simulink library "cool_simple_retOnly_std"  (R2016a)
settings: Solver=VariableStepAuto  StartTime=0.0  StopTime=10.0  RelTol=1e-3
undefined symbols (not defined in the file): sMP
settings Model: Creator=JEKREMS  LastModifiedBy=JEKREMS
settings GRTTargetCC: GeneratePreprocessorConditionals=Use local settings

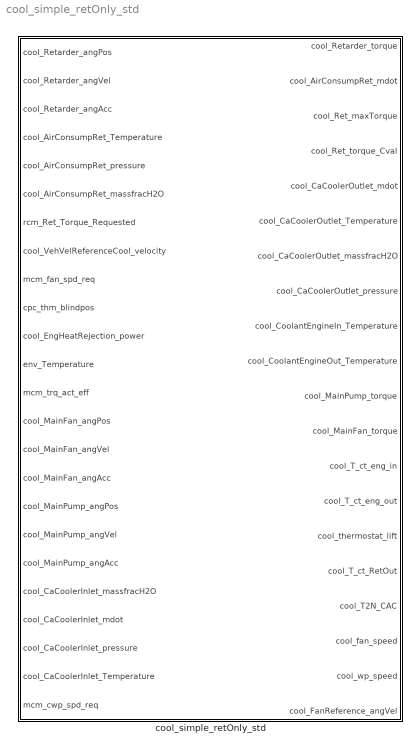
== system cool_simple_retOnly_std ==
  cool_simple_retOnly_std : Subsystem  mask{prm_to_disp=[1..10], sfcnParam1=sMP.phys.cool.fan.x_fan_rpm_schlepp, sfcnParam2=sMP.phys.cool.fan.y_fan_M_schlepp, sfcnParam3=sMP.phys.cool.out.cool_CaCoolerOutlet_Temperature, sfcnParam4=sMP.phys.cool.out.cool_CoolantEngineIn_Temperature, sfcnParam5=sMP.phys.cool.out.cool_CoolantEngineOut_Temperature, sfcnParam6=sMP.phys.cool.out.cool_T2N_CAC, sfcnParam7=sMP.phys.cool.out.cool_T_ct_RetOut, sfcnParam8=sMP.phys.cool.out.cool_T_ct_eng_in, sfcnParam9=sMP.phys.cool.out.cool_T_ct_eng_out, sfcnParam10=sMP.phys.cool.ret.x_ret_rpm, sfcnParam11=sMP.phys.cool.ret.x_ret_rpm_schlepp, sfcnParam12=sMP.phys.cool.ret.y_ret_M_max, sfcnParam13=sMP.phys.cool.ret.y_ret_M_schlepp}
      mask prompts: prm_to_disp "Display S-function Parameters:"; sfcnParam1 "fan_x_fan_rpm_schlepp:"; sfcnParam2 "fan_y_fan_M_schlepp:"; sfcnParam3 "out_cool_CaCoolerOutlet_Temperature:"; sfcnParam4 "out_cool_CoolantEngineIn_Temperature:"; sfcnParam5 "out_cool_CoolantEngineOut_Temperature:"; sfcnParam6 "out_cool_T2N_CAC:"; sfcnParam7 "out_cool_T_ct_RetOut:"; sfcnParam8 "out_cool_T_ct_eng_in:"; sfcnParam9 "out_cool_T_ct_eng_out:"; sfcnParam10 "ret_x_ret_rpm:"; sfcnParam11 "ret_x_ret_rpm_schlepp:"; sfcnParam12 "ret_y_ret_M_max:"; sfcnParam13 "ret_y_ret_M_schlepp:"
      mask help: Simulink:masks:GenSFuncDesc_MD
      mask Help: eval('feval(''rtwprivate'',''rtwhelpview'',''rtw_sfcn_block'')');
      mask TypeOptions prm_to_disp: [1..10] | [11..13]
      mask Callback prm_to_disp: slmaskprmdispcntrl(gcbh)

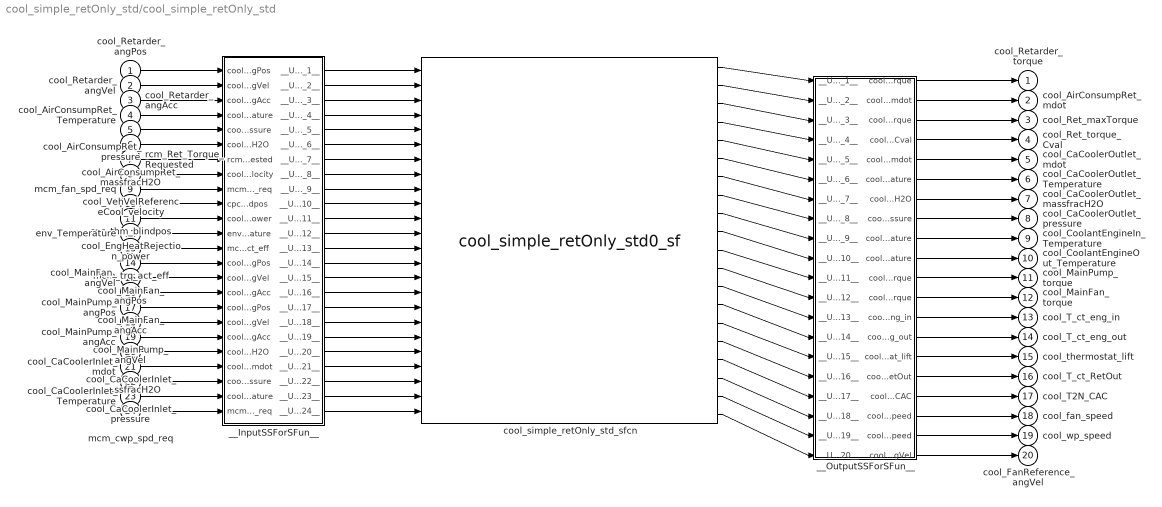
== system cool_simple_retOnly_std/cool_simple_retOnly_std ==
  cool_Retarder_angPos : Inport
  cool_Retarder_angVel : Inport  Port=2
  cool_Retarder_angAcc : Inport  Port=3
  cool_AirConsumpRet_Temperature : Inport  Port=4
  cool_AirConsumpRet_pressure : Inport  Port=5
  cool_AirConsumpRet_massfracH2O : Inport  Port=6
  rcm_Ret_Torque_Requested : Inport  Port=7
  cool_VehVelReferenceCool_velocity : Inport  Port=8
  mcm_fan_spd_req : Inport  Port=9
  cpc_thm_blindpos : Inport  Port=10
  cool_EngHeatRejection_power : Inport  Port=11
  env_Temperature : Inport  Port=12
  mcm_trq_act_eff : Inport  Port=13
  cool_MainFan_angPos : Inport  Port=14
  cool_MainFan_angVel : Inport  Port=15
  cool_MainFan_angAcc : Inport  Port=16
  cool_MainPump_angPos : Inport  Port=17
  cool_MainPump_angVel : Inport  Port=18
  cool_MainPump_angAcc : Inport  Port=19
  cool_CaCoolerInlet_massfracH2O : Inport  Port=20
  cool_CaCoolerInlet_mdot : Inport  Port=21
  cool_CaCoolerInlet_pressure : Inport  Port=22
  cool_CaCoolerInlet_Temperature : Inport  Port=23
  mcm_cwp_spd_req : Inport  Port=24
  __InputSSForSFun__ : Subsystem
  __OutputSSForSFun__ : Subsystem
  cool_simple_retOnly_std_sfcn : S-Function  FunctionName=cool_simple_retOnly_std0_sf  Parameters=sfcnParam1, sfcnParam2, sfcnParam3, sfcnParam4, sfcnParam5, sfcnParam6, sfcnParam7, sfcnParam8, sfcnParam9, sfcnParam10, sfcnParam11, sfcnParam12, sfcnParam13  SFunctionModules=""  SFunctionDeploymentMode=off  EnableBusSupport=off  mask{rtw_sf_name=cool_simple_retOnly_std0_sf, showVar=off, prm_to_disp=[1..10], sfcnParam1=sfcnParam1, sfcnParam2=sfcnParam2, sfcnParam3=sfcnParam3, sfcnParam4=sfcnParam4, sfcnParam5=sfcnParam5, sfcnParam6=sfcnParam6, sfcnParam7=sfcnParam7, sfcnParam8=sfcnParam8, sfcnParam9=sfcnParam9, sfcnParam10=sfcnParam10, sfcnParam11=sfcnParam11, sfcnParam12=sfcnParam12, sfcnParam13=sfcnParam13}
      mask prompts: rtw_sf_name "Simulink:masks:GenSFuncName_MP"; showVar "Simulink:masks:GenSFuncShowModuleList_MP"; prm_to_disp "Display S-function Parameters:"; sfcnParam1 "sMP_phys_cool_fan_x_fan_rpm_schlepp:"; sfcnParam2 "sMP_phys_cool_fan_y_fan_M_schlepp:"; sfcnParam3 "sMP_phys_cool_out_cool_CaCoolerOutlet_Temperature:"; sfcnParam4 "sMP_phys_cool_out_cool_CoolantEngineIn_Temperature:"; sfcnParam5 "sMP_phys_cool_out_cool_CoolantEngineOut_Temperature:"; sfcnParam6 "sMP_phys_cool_out_cool_T2N_CAC:"; sfcnParam7 "sMP_phys_cool_out_cool_T_ct_RetOut:"; sfcnParam8 "sMP_phys_cool_out_cool_T_ct_eng_in:"; sfcnParam9 "sMP_phys_cool_out_cool_T_ct_eng_out:"; sfcnParam10 "sMP_phys_cool_ret_x_ret_rpm:"; sfcnParam11 "sMP_phys_cool_ret_x_ret_rpm_schlepp:"; sfcnParam12 "sMP_phys_cool_ret_y_ret_M_max:"; sfcnParam13 "sMP_phys_cool_ret_y_ret_M_schlepp:"
      mask help: Simulink:masks:GenSFuncDesc_MD
      mask init:
      | displist = '';
      | if ~strcmp(get_param(gcb, 'FunctionName'), rtw_sf_name);
      |   set_param(gcb, 'FunctionName', rtw_sf_name);
      | end
      | % Check if we are generating code
      | rtw_mode = false;
      | if strcmpi(get_param(bdroot(gcb),'SimulationStatus'),'Initializing')
      | 	rtw_mode = strcmpi(get_param(bdroot(gcb),'BuildingRTWCode'),'on') && ...
      | 		~strcmpi(get_param(bdroot(gcb),'TargetStyle'),'SimulationTarget');
      | end
      | if showVar || rtw_mode
      | 	if exist('rtwsfunc') == 2 | exist('rtwsfunc') == 6
      | 		tmplist = rtwsfunc(rtw_sf_name,gcb);
      | 		tmplist = DAStudio.message('Simulink:masks:GenSFuncListOfModules_IC', tmplist);
      | 	elseif showVar
      | 		tmplist1 = DAStudio.message('Simulink:masks:GenSFuncListOfModules_IC', '');
      |         tmplist2 = DAStudio.message('Simulink:masks:GenSFuncNotLicensed_IC');
      |         tmplist = [tmplist1 tmplist2];
      |  	end
      | end
      | if showVar
      |   displist = tmplist;
      | end
      settings: CopyFcn=|
      | if ~strcmp(get_param(gcb,'Linkstatus'),'none') && ...
      | ~strcmp(get_param(gcb,'Linkstatus'),'implicit')
      |   set_param(gcb,'LinkStatus','none');
      | end
      mask Help: eval('feval(''rtwprivate'',''rtwhelpview'',''rtw_sfcn_block'')');
      mask TypeOptions prm_to_disp: [1..10] | [11..13]
      mask Callback prm_to_disp: slmaskprmdispcntrl(gcbh)
      mask Display:
      | port_label('input',1,'cool_Retarder_angPos');
      | port_label('input',2,'cool_Retarder_angVel');
      | port_label('input',3,'cool_Retarder_angAcc');
      | port_label('input',4,'cool_AirConsumpRet_Temperature');
      | port_label('input',5,'cool_AirConsumpRet_pressure');
      | port_label('input',6,'cool_AirConsumpRet_massfracH2O');
      | port_label('input',7,'rcm_Ret_Torque_Requested');
      | port_label('input',8,'cool_VehVelReferenceCool_velocity');
      | port_label('input',9,'mcm_fan_spd_req');
      | port_label('input',10,'cpc_thm_blindpos');
      | port_label('input',11,'cool_EngHeatRejection_power');
      | port_label('input',12,'env_Temperature');
      | port_label('input',13,'mcm_trq_act_eff');
      | port_label('input',14,'cool_MainFan_angPos');
      | port_label('input',15,'cool_MainFan_angVel');
      | port_label('input',16,'cool_MainFan_angAcc');
      | port_label('input',17,'cool_MainPump_angPos');
      | port_label('input',18,'cool_MainPump_angVel');
      | port_label('input',19,'cool_MainPump_angAcc');
      | port_label('input',20,'cool_CaCoolerInlet_massfracH2O');
      | port_label('input',21,'cool_CaCoolerInlet_mdot');
      | port_label('input',22,'cool_CaCoolerInlet_pressure');
      | port_label('input',23,'cool_CaCoolerInlet_Temperature');
      | port_label('input',24,'mcm_cwp_spd_req');
      | port_label('output',1,'cool_Retarder_torque');
      | port_label('output',2,'cool_AirConsumpRet_mdot');
      | port_label('output',3,'cool_Ret_maxTorque');
      | port_label('output',4,'cool_Ret_torque_Cval');
      | port_label('output',5,'cool_CaCoolerOutlet_mdot');
      | port_label('output',6,'cool_CaCoolerOutlet_Temperature');
      | port_label('output',7,'cool_CaCoolerOutlet_massfracH2O');
      | port_label('output',8,'cool_CaCoolerOutlet_pressure');
      | port_label('output',9,'cool_CoolantEngineIn_Temperature');
      | port_label('output',10,'cool_CoolantEngineOut_Temperature');
      | port_label('output',11,'cool_MainPump_torque');
      | port_label('output',12,'cool_MainFan_torque');
      | port_label('output',13,'cool_T_ct_eng_in');
      | port_label('output',14,'cool_T_ct_eng_out');
      | port_label('output',15,'cool_thermostat_lift');
      | port_label('output',16,'cool_T_ct_RetOut');
      | port_label('output',17,'cool_T2N_CAC');
      | port_label('output',18,'cool_fan_speed');
      | port_label('output',19,'cool_wp_speed');
      | port_label('output',20,'cool_FanReference_angVel');
  cool_Retarder_torque : Outport
  cool_AirConsumpRet_mdot : Outport  Port=2
  cool_Ret_maxTorque : Outport  Port=3
  cool_Ret_torque_Cval : Outport  Port=4
  cool_CaCoolerOutlet_mdot : Outport  Port=5
  cool_CaCoolerOutlet_Temperature : Outport  Port=6
  cool_CaCoolerOutlet_massfracH2O : Outport  Port=7
  cool_CaCoolerOutlet_pressure : Outport  Port=8
  cool_CoolantEngineIn_Temperature : Outport  Port=9
  cool_CoolantEngineOut_Temperature : Outport  Port=10
  cool_MainPump_torque : Outport  Port=11
  cool_MainFan_torque : Outport  Port=12
  cool_T_ct_eng_in : Outport  Port=13
  cool_T_ct_eng_out : Outport  Port=14
  cool_thermostat_lift : Outport  Port=15
  cool_T_ct_RetOut : Outport  Port=16
  cool_T2N_CAC : Outport  Port=17
  cool_fan_speed : Outport  Port=18
  cool_wp_speed : Outport  Port=19
  cool_FanReference_angVel : Outport  Port=20
  wires:
  __OutputSSForSFun__/20(cool_FanReference_angVel) -> cool_FanReference_angVel/1
  __OutputSSForSFun__/19(cool_wp_speed) -> cool_wp_speed/1
  __OutputSSForSFun__/18(cool_fan_speed) -> cool_fan_speed/1
  __OutputSSForSFun__/17(cool_T2N_CAC) -> cool_T2N_CAC/1
  __OutputSSForSFun__/16(cool_T_ct_RetOut) -> cool_T_ct_RetOut/1
  __OutputSSForSFun__/15(cool_thermostat_lift) -> cool_thermostat_lift/1
  __OutputSSForSFun__/14(cool_T_ct_eng_out) -> cool_T_ct_eng_out/1
  __OutputSSForSFun__/13(cool_T_ct_eng_in) -> cool_T_ct_eng_in/1
  __OutputSSForSFun__/12(cool_MainFan_torque) -> cool_MainFan_torque/1
  __OutputSSForSFun__/11(cool_MainPump_torque) -> cool_MainPump_torque/1
  __OutputSSForSFun__/10(cool_CoolantEngineOut_Temperature) -> cool_CoolantEngineOut_Temperature/1
  __OutputSSForSFun__/9(cool_CoolantEngineIn_Temperature) -> cool_CoolantEngineIn_Temperature/1
  __OutputSSForSFun__/8(cool_CaCoolerOutlet_pressure) -> cool_CaCoolerOutlet_pressure/1
  __OutputSSForSFun__/7(cool_CaCoolerOutlet_massfracH2O) -> cool_CaCoolerOutlet_massfracH2O/1
  __OutputSSForSFun__/6(cool_CaCoolerOutlet_Temperature) -> cool_CaCoolerOutlet_Temperature/1
  __OutputSSForSFun__/5(cool_CaCoolerOutlet_mdot) -> cool_CaCoolerOutlet_mdot/1
  __OutputSSForSFun__/4(cool_Ret_torque_Cval) -> cool_Ret_torque_Cval/1
  __OutputSSForSFun__/3(cool_Ret_maxTorque) -> cool_Ret_maxTorque/1
  __OutputSSForSFun__/2(cool_AirConsumpRet_mdot) -> cool_AirConsumpRet_mdot/1
  __OutputSSForSFun__/1(cool_Retarder_torque) -> cool_Retarder_torque/1
  cool_simple_retOnly_std_sfcn/20 -> __OutputSSForSFun__/20(__UniqueInportName__20__)
  cool_simple_retOnly_std_sfcn/19 -> __OutputSSForSFun__/19(__UniqueInportName__19__)
  cool_simple_retOnly_std_sfcn/18 -> __OutputSSForSFun__/18(__UniqueInportName__18__)
  cool_simple_retOnly_std_sfcn/17 -> __OutputSSForSFun__/17(__UniqueInportName__17__)
  cool_simple_retOnly_std_sfcn/16 -> __OutputSSForSFun__/16(__UniqueInportName__16__)
  cool_simple_retOnly_std_sfcn/15 -> __OutputSSForSFun__/15(__UniqueInportName__15__)
  cool_simple_retOnly_std_sfcn/14 -> __OutputSSForSFun__/14(__UniqueInportName__14__)
  cool_simple_retOnly_std_sfcn/13 -> __OutputSSForSFun__/13(__UniqueInportName__13__)
  cool_simple_retOnly_std_sfcn/12 -> __OutputSSForSFun__/12(__UniqueInportName__12__)
  cool_simple_retOnly_std_sfcn/11 -> __OutputSSForSFun__/11(__UniqueInportName__11__)
  cool_simple_retOnly_std_sfcn/10 -> __OutputSSForSFun__/10(__UniqueInportName__10__)
  cool_simple_retOnly_std_sfcn/9 -> __OutputSSForSFun__/9(__UniqueInportName__9__)
  cool_simple_retOnly_std_sfcn/8 -> __OutputSSForSFun__/8(__UniqueInportName__8__)
  cool_simple_retOnly_std_sfcn/7 -> __OutputSSForSFun__/7(__UniqueInportName__7__)
  cool_simple_retOnly_std_sfcn/6 -> __OutputSSForSFun__/6(__UniqueInportName__6__)
  cool_simple_retOnly_std_sfcn/5 -> __OutputSSForSFun__/5(__UniqueInportName__5__)
  cool_simple_retOnly_std_sfcn/4 -> __OutputSSForSFun__/4(__UniqueInportName__4__)
  cool_simple_retOnly_std_sfcn/3 -> __OutputSSForSFun__/3(__UniqueInportName__3__)
  cool_simple_retOnly_std_sfcn/2 -> __OutputSSForSFun__/2(__UniqueInportName__2__)
  cool_simple_retOnly_std_sfcn/1 -> __OutputSSForSFun__/1(__UniqueInportName__1__)
  __InputSSForSFun__/24(__UniqueOutportName__24__) -> cool_simple_retOnly_std_sfcn/24
  __InputSSForSFun__/23(__UniqueOutportName__23__) -> cool_simple_retOnly_std_sfcn/23
  __InputSSForSFun__/22(__UniqueOutportName__22__) -> cool_simple_retOnly_std_sfcn/22
  __InputSSForSFun__/21(__UniqueOutportName__21__) -> cool_simple_retOnly_std_sfcn/21
  __InputSSForSFun__/20(__UniqueOutportName__20__) -> cool_simple_retOnly_std_sfcn/20
  __InputSSForSFun__/19(__UniqueOutportName__19__) -> cool_simple_retOnly_std_sfcn/19
  __InputSSForSFun__/18(__UniqueOutportName__18__) -> cool_simple_retOnly_std_sfcn/18
  __InputSSForSFun__/17(__UniqueOutportName__17__) -> cool_simple_retOnly_std_sfcn/17
  __InputSSForSFun__/16(__UniqueOutportName__16__) -> cool_simple_retOnly_std_sfcn/16
  __InputSSForSFun__/15(__UniqueOutportName__15__) -> cool_simple_retOnly_std_sfcn/15
  __InputSSForSFun__/14(__UniqueOutportName__14__) -> cool_simple_retOnly_std_sfcn/14
  __InputSSForSFun__/13(__UniqueOutportName__13__) -> cool_simple_retOnly_std_sfcn/13
  __InputSSForSFun__/12(__UniqueOutportName__12__) -> cool_simple_retOnly_std_sfcn/12
  __InputSSForSFun__/11(__UniqueOutportName__11__) -> cool_simple_retOnly_std_sfcn/11
  __InputSSForSFun__/10(__UniqueOutportName__10__) -> cool_simple_retOnly_std_sfcn/10
  __InputSSForSFun__/9(__UniqueOutportName__9__) -> cool_simple_retOnly_std_sfcn/9
  __InputSSForSFun__/8(__UniqueOutportName__8__) -> cool_simple_retOnly_std_sfcn/8
  __InputSSForSFun__/7(__UniqueOutportName__7__) -> cool_simple_retOnly_std_sfcn/7
  __InputSSForSFun__/6(__UniqueOutportName__6__) -> cool_simple_retOnly_std_sfcn/6
  __InputSSForSFun__/5(__UniqueOutportName__5__) -> cool_simple_retOnly_std_sfcn/5
  __InputSSForSFun__/4(__UniqueOutportName__4__) -> cool_simple_retOnly_std_sfcn/4
  __InputSSForSFun__/3(__UniqueOutportName__3__) -> cool_simple_retOnly_std_sfcn/3
  __InputSSForSFun__/2(__UniqueOutportName__2__) -> cool_simple_retOnly_std_sfcn/2
  __InputSSForSFun__/1(__UniqueOutportName__1__) -> cool_simple_retOnly_std_sfcn/1
  mcm_cwp_spd_req/1 -> __InputSSForSFun__/24(mcm_cwp_spd_req)
  cool_CaCoolerInlet_Temperature/1 -> __InputSSForSFun__/23(cool_CaCoolerInlet_Temperature)
  cool_CaCoolerInlet_pressure/1 -> __InputSSForSFun__/22(cool_CaCoolerInlet_pressure)
  cool_CaCoolerInlet_mdot/1 -> __InputSSForSFun__/21(cool_CaCoolerInlet_mdot)
  cool_CaCoolerInlet_massfracH2O/1 -> __InputSSForSFun__/20(cool_CaCoolerInlet_massfracH2O)
  cool_MainPump_angAcc/1 -> __InputSSForSFun__/19(cool_MainPump_angAcc)
  cool_MainPump_angVel/1 -> __InputSSForSFun__/18(cool_MainPump_angVel)
  cool_MainPump_angPos/1 -> __InputSSForSFun__/17(cool_MainPump_angPos)
  cool_MainFan_angAcc/1 -> __InputSSForSFun__/16(cool_MainFan_angAcc)
  cool_MainFan_angVel/1 -> __InputSSForSFun__/15(cool_MainFan_angVel)
  cool_MainFan_angPos/1 -> __InputSSForSFun__/14(cool_MainFan_angPos)
  mcm_trq_act_eff/1 -> __InputSSForSFun__/13(mcm_trq_act_eff)
  env_Temperature/1 -> __InputSSForSFun__/12(env_Temperature)
  cool_EngHeatRejection_power/1 -> __InputSSForSFun__/11(cool_EngHeatRejection_power)
  cpc_thm_blindpos/1 -> __InputSSForSFun__/10(cpc_thm_blindpos)
  mcm_fan_spd_req/1 -> __InputSSForSFun__/9(mcm_fan_spd_req)
  cool_VehVelReferenceCool_velocity/1 -> __InputSSForSFun__/8(cool_VehVelReferenceCool_velocity)
  rcm_Ret_Torque_Requested/1 -> __InputSSForSFun__/7(rcm_Ret_Torque_Requested)
  cool_AirConsumpRet_massfracH2O/1 -> __InputSSForSFun__/6(cool_AirConsumpRet_massfracH2O)
  cool_AirConsumpRet_pressure/1 -> __InputSSForSFun__/5(cool_AirConsumpRet_pressure)
  cool_AirConsumpRet_Temperature/1 -> __InputSSForSFun__/4(cool_AirConsumpRet_Temperature)
  cool_Retarder_angAcc/1 -> __InputSSForSFun__/3(cool_Retarder_angAcc)
  cool_Retarder_angVel/1 -> __InputSSForSFun__/2(cool_Retarder_angVel)
  cool_Retarder_angPos/1 -> __InputSSForSFun__/1(cool_Retarder_angPos)

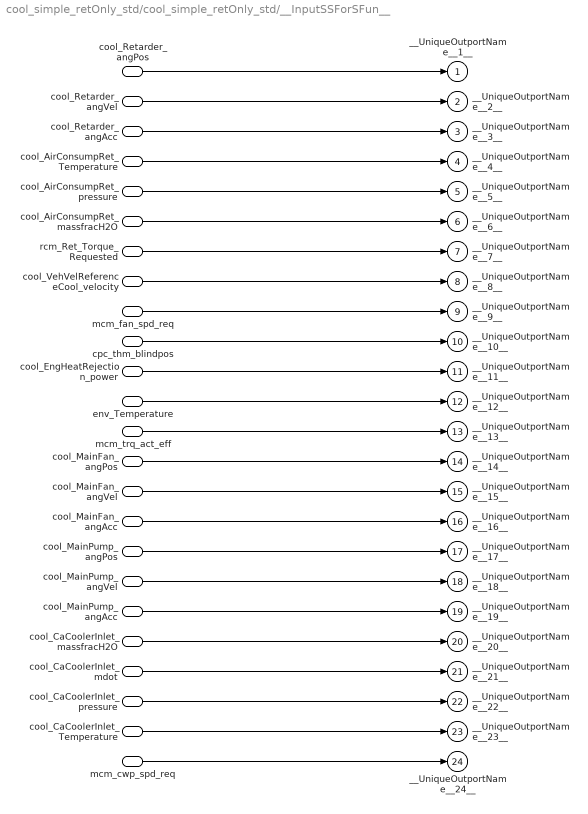
== system cool_simple_retOnly_std/cool_simple_retOnly_std/__InputSSForSFun__ ==
  cool_Retarder_angPos : Inport
  cool_Retarder_angVel : Inport  Port=2
  cool_Retarder_angAcc : Inport  Port=3
  cool_AirConsumpRet_Temperature : Inport  Port=4
  cool_AirConsumpRet_pressure : Inport  Port=5
  cool_AirConsumpRet_massfracH2O : Inport  Port=6
  rcm_Ret_Torque_Requested : Inport  Port=7
  cool_VehVelReferenceCool_velocity : Inport  Port=8
  mcm_fan_spd_req : Inport  Port=9
  cpc_thm_blindpos : Inport  Port=10
  cool_EngHeatRejection_power : Inport  Port=11
  env_Temperature : Inport  Port=12
  mcm_trq_act_eff : Inport  Port=13
  cool_MainFan_angPos : Inport  Port=14
  cool_MainFan_angVel : Inport  Port=15
  cool_MainFan_angAcc : Inport  Port=16
  cool_MainPump_angPos : Inport  Port=17
  cool_MainPump_angVel : Inport  Port=18
  cool_MainPump_angAcc : Inport  Port=19
  cool_CaCoolerInlet_massfracH2O : Inport  Port=20
  cool_CaCoolerInlet_mdot : Inport  Port=21
  cool_CaCoolerInlet_pressure : Inport  Port=22
  cool_CaCoolerInlet_Temperature : Inport  Port=23
  mcm_cwp_spd_req : Inport  Port=24
  __UniqueOutportName__1__ : Outport
  __UniqueOutportName__2__ : Outport  Port=2
  __UniqueOutportName__3__ : Outport  Port=3
  __UniqueOutportName__4__ : Outport  Port=4
  __UniqueOutportName__5__ : Outport  Port=5
  __UniqueOutportName__6__ : Outport  Port=6
  __UniqueOutportName__7__ : Outport  Port=7
  __UniqueOutportName__8__ : Outport  Port=8
  __UniqueOutportName__9__ : Outport  Port=9
  __UniqueOutportName__10__ : Outport  Port=10
  __UniqueOutportName__11__ : Outport  Port=11
  __UniqueOutportName__12__ : Outport  Port=12
  __UniqueOutportName__13__ : Outport  Port=13
  __UniqueOutportName__14__ : Outport  Port=14
  __UniqueOutportName__15__ : Outport  Port=15
  __UniqueOutportName__16__ : Outport  Port=16
  __UniqueOutportName__17__ : Outport  Port=17
  __UniqueOutportName__18__ : Outport  Port=18
  __UniqueOutportName__19__ : Outport  Port=19
  __UniqueOutportName__20__ : Outport  Port=20
  __UniqueOutportName__21__ : Outport  Port=21
  __UniqueOutportName__22__ : Outport  Port=22
  __UniqueOutportName__23__ : Outport  Port=23
  __UniqueOutportName__24__ : Outport  Port=24
  wires:
  mcm_cwp_spd_req/1 -> __UniqueOutportName__24__/1
  cool_CaCoolerInlet_Temperature/1 -> __UniqueOutportName__23__/1
  cool_CaCoolerInlet_pressure/1 -> __UniqueOutportName__22__/1
  cool_CaCoolerInlet_mdot/1 -> __UniqueOutportName__21__/1
  cool_CaCoolerInlet_massfracH2O/1 -> __UniqueOutportName__20__/1
  cool_MainPump_angAcc/1 -> __UniqueOutportName__19__/1
  cool_MainPump_angVel/1 -> __UniqueOutportName__18__/1
  cool_MainPump_angPos/1 -> __UniqueOutportName__17__/1
  cool_MainFan_angAcc/1 -> __UniqueOutportName__16__/1
  cool_MainFan_angVel/1 -> __UniqueOutportName__15__/1
  cool_MainFan_angPos/1 -> __UniqueOutportName__14__/1
  mcm_trq_act_eff/1 -> __UniqueOutportName__13__/1
  env_Temperature/1 -> __UniqueOutportName__12__/1
  cool_EngHeatRejection_power/1 -> __UniqueOutportName__11__/1
  cpc_thm_blindpos/1 -> __UniqueOutportName__10__/1
  mcm_fan_spd_req/1 -> __UniqueOutportName__9__/1
  cool_VehVelReferenceCool_velocity/1 -> __UniqueOutportName__8__/1
  rcm_Ret_Torque_Requested/1 -> __UniqueOutportName__7__/1
  cool_AirConsumpRet_massfracH2O/1 -> __UniqueOutportName__6__/1
  cool_AirConsumpRet_pressure/1 -> __UniqueOutportName__5__/1
  cool_AirConsumpRet_Temperature/1 -> __UniqueOutportName__4__/1
  cool_Retarder_angAcc/1 -> __UniqueOutportName__3__/1
  cool_Retarder_angVel/1 -> __UniqueOutportName__2__/1
  cool_Retarder_angPos/1 -> __UniqueOutportName__1__/1

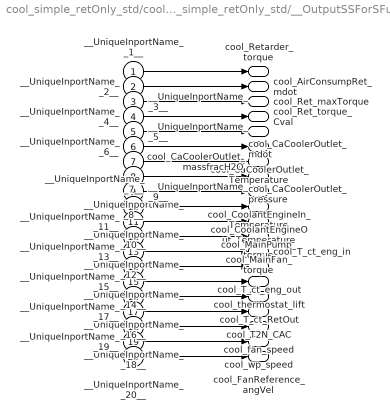
== system cool_simple_retOnly_std/cool_simple_retOnly_std/__OutputSSForSFun__ ==
  __UniqueInportName__1__ : Inport
  __UniqueInportName__2__ : Inport  Port=2
  __UniqueInportName__3__ : Inport  Port=3
  __UniqueInportName__4__ : Inport  Port=4
  __UniqueInportName__5__ : Inport  Port=5
  __UniqueInportName__6__ : Inport  Port=6
  __UniqueInportName__7__ : Inport  Port=7
  __UniqueInportName__8__ : Inport  Port=8
  __UniqueInportName__9__ : Inport  Port=9
  __UniqueInportName__10__ : Inport  Port=10
  __UniqueInportName__11__ : Inport  Port=11
  __UniqueInportName__12__ : Inport  Port=12
  __UniqueInportName__13__ : Inport  Port=13
  __UniqueInportName__14__ : Inport  Port=14
  __UniqueInportName__15__ : Inport  Port=15
  __UniqueInportName__16__ : Inport  Port=16
  __UniqueInportName__17__ : Inport  Port=17
  __UniqueInportName__18__ : Inport  Port=18
  __UniqueInportName__19__ : Inport  Port=19
  __UniqueInportName__20__ : Inport  Port=20
  cool_Retarder_torque : Outport
  cool_AirConsumpRet_mdot : Outport  Port=2
  cool_Ret_maxTorque : Outport  Port=3
  cool_Ret_torque_Cval : Outport  Port=4
  cool_CaCoolerOutlet_mdot : Outport  Port=5
  cool_CaCoolerOutlet_Temperature : Outport  Port=6
  cool_CaCoolerOutlet_massfracH2O : Outport  Port=7
  cool_CaCoolerOutlet_pressure : Outport  Port=8
  cool_CoolantEngineIn_Temperature : Outport  Port=9
  cool_CoolantEngineOut_Temperature : Outport  Port=10
  cool_MainPump_torque : Outport  Port=11
  cool_MainFan_torque : Outport  Port=12
  cool_T_ct_eng_in : Outport  Port=13
  cool_T_ct_eng_out : Outport  Port=14
  cool_thermostat_lift : Outport  Port=15
  cool_T_ct_RetOut : Outport  Port=16
  cool_T2N_CAC : Outport  Port=17
  cool_fan_speed : Outport  Port=18
  cool_wp_speed : Outport  Port=19
  cool_FanReference_angVel : Outport  Port=20
  wires:
  __UniqueInportName__20__/1 -> cool_FanReference_angVel/1
  __UniqueInportName__19__/1 -> cool_wp_speed/1
  __UniqueInportName__18__/1 -> cool_fan_speed/1
  __UniqueInportName__17__/1 -> cool_T2N_CAC/1
  __UniqueInportName__16__/1 -> cool_T_ct_RetOut/1
  __UniqueInportName__15__/1 -> cool_thermostat_lift/1
  __UniqueInportName__14__/1 -> cool_T_ct_eng_out/1
  __UniqueInportName__13__/1 -> cool_T_ct_eng_in/1
  __UniqueInportName__12__/1 -> cool_MainFan_torque/1
  __UniqueInportName__11__/1 -> cool_MainPump_torque/1
  __UniqueInportName__10__/1 -> cool_CoolantEngineOut_Temperature/1
  __UniqueInportName__9__/1 -> cool_CoolantEngineIn_Temperature/1
  __UniqueInportName__8__/1 -> cool_CaCoolerOutlet_pressure/1
  __UniqueInportName__7__/1 -> cool_CaCoolerOutlet_massfracH2O/1
  __UniqueInportName__6__/1 -> cool_CaCoolerOutlet_Temperature/1
  __UniqueInportName__5__/1 -> cool_CaCoolerOutlet_mdot/1
  __UniqueInportName__4__/1 -> cool_Ret_torque_Cval/1
  __UniqueInportName__3__/1 -> cool_Ret_maxTorque/1
  __UniqueInportName__2__/1 -> cool_AirConsumpRet_mdot/1
  __UniqueInportName__1__/1 -> cool_Retarder_torque/1
